simulink library "Lib_Turbo_HeatXchang_TMATS"  (R2013b)
settings: Solver=ode45  StartTime=0.0  StopTime=10.0  RelTol=1e-3
libraries: Lib_Thermo_Temp2Enth_TMATS x4, Lib_Thermo_Enth2Temp_TMATS x2, Lib_Solve_DataOut_TMATS x1
Description:
  | Thomas Modules
settings Model: Creator=jwchapm2  LastModifiedBy=jwchapm2

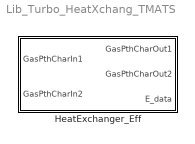
== system Lib_Turbo_HeatXchang_TMATS ==
  HeatExchanger_Eff : Subsystem  mask(T-MATS: HeatExchanger_Eff Library Block){dP1_M=0.005, dP2_M=0.005, E_M=0.5, iDesign_M=2, dQDes_M=1000, FVar_M='iDesScalars.mat', SVar_M=gcb, ENm_M='_E'}
      mask prompts: dP1_M "dP1_M - Delta Pressure for input 1 [frac lost]"; dP2_M "dP2_M - Delta Pressure for input 2 [frac lost]"; E_M "E_M - heat transfer effectiveness [frac]"; iDesign_M "iDesign_M - Design fork (0 - Enable iDes, 1 - Use iDes E, 2 - Use Input E)"; dQDes_M "dQDes_M - Delta Energy Design [BTU/sec]"; FVar_M "FVar_M - File name for iDes Variables"; SVar_M "SVar_M - iDes Variable Surname"; ENm_M "ENm_M - iDes Effectiveness variable name"
      mask help: This block simulates the performance of a heat exchanger using effectiveness-NTU method based on heat transfer efffectiveness, E.
      mask init:
      | if iDesign_M == 1
      |     load(FVar_M);
      |     E_M = eval(strcat(stripchar_TMATS(SVar_M),ENm_M));
      | end
      mask Help: web(which('Turbo_TMATS_HtXferEff.html'),'-helpbrowser')
      mask Callback iDesign_M:
      | MSK_SEC_Enables_Ides_TMATS('iDesign_M',[3],'G1')
      | MSK_SEC_Enables_Ides_TMATS('iDesign_M',[5],'G2')
      | MSK_SEC_Enables_Ides_TMATS('iDesign_M',[6 7 8],'G3')

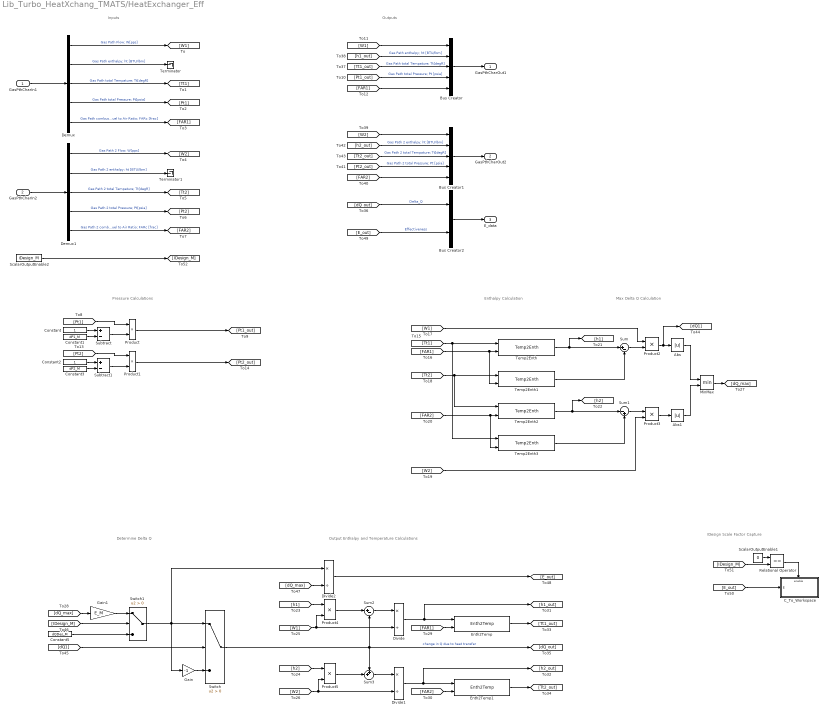
== system Lib_Turbo_HeatXchang_TMATS/HeatExchanger_Eff ==
  note: Pressure Calculations
  note: Max Delta Q Calculation
  note: Output Enthalpy and Temperature Calculations
  note: Outputs
  note: Inputs
  note: IDesign Scale Factor Capture
  note: Enthalpy Calculation
  note: Determine Delta Q
  GasPthCharIn1 : Inport
  GasPthCharIn2 : Inport  Port=2
  Abs : Abs
  Abs1 : Abs
  Bus Creator : BusCreator  Inputs=5
  Bus Creator1 : BusCreator  Inputs=5
  Bus Creator2 : BusCreator  Inputs=2
  C_To_Workspace : Subsystem
  Constant : Constant
  Constant1 : Constant  Value=dP1_M
  Constant2 : Constant
  Constant3 : Constant  Value=dP2_M
  Constant5 : Constant  Value=dQDes_M
  Demux : Demux  Outputs=5
  Demux1 : Demux  Outputs=5
  Divide : Product  Inputs=*/
  Divide1 : Product  Inputs=*/
  Divide2 : Product  Inputs=*/
  Enth2Temp : Lib_Thermo_Enth2Temp_TMATS/Enth2Temp
  Enth2Temp1 : Lib_Thermo_Enth2Temp_TMATS/Enth2Temp
  Gain : Gain  Gain=-1
  Gain1 : Gain  Gain=E_M
  MinMax : MinMax  Inputs=2
  Product : Product  RndMeth=Zero
  Product1 : Product  RndMeth=Zero
  Product{2..5} (4 alike) : Product
  Relational Operator : RelationalOperator  Operator===  OutDataTypeStr=boolean
  ScalarOutputEnable1 : Constant  Value=0
  ScalarOutputEnable2 : Constant  Value=iDesign_M
  Subtract : Sum  Inputs=+-
  Subtract1 : Sum  Inputs=+-
  Sum : Sum  Inputs=|+-
  Sum1 : Sum  Inputs=|-+
  Sum2 : Sum  Inputs=|+-
  Sum3 : Sum  Inputs=++|
  Switch : Switch  Criteria=u2 > Threshold
  Switch1 : Switch  Criteria=u2 > Threshold
  Temp2Enth{,1..3} (4 alike) : Lib_Thermo_Temp2Enth_TMATS/Temp2Enth
  Terminator : Terminator
  Terminator1 : Terminator
  GasPthCharOut1 : Outport
  GasPthCharOut2 : Outport  Port=2
  E_data : Outport  Port=3
  wires:
  Constant/1 -> Subtract/1
  Constant1/1 -> Subtract/2
  Demux/1 -> [W1]  "Gas Path Flow; W[pps]"
  Demux/5 -> [FAR1]  "Gas Path combusted Fuel to Air Ratio; FARc [frac]"
  Demux/3 -> [Tt1]  "Gas Path total Tempature; Tt[degR]"
  GasPthCharIn1/1 -> Demux/1
  Bus Creator/1 -> GasPthCharOut1/1
  Product/1 -> [Pt1_out]
  Demux/4 -> [Pt1]  "Gas Path total Pressure; Pt[psia]"
  Subtract/1 -> Product/2
  Demux/2 -> Terminator/1  "Gas Path enthalpy; ht [BTU/lbm]"
  Demux1/1 -> [W2]  "Gas Path 2 Flow; W[pps]"
  Demux1/5 -> [FAR2]  "Gas Path 2 combusted Fuel to Air Ratio; FARc [frac]"
  Demux1/3 -> [Tt2]  "Gas Path 2 total Tempature; Tt[degR]"
  GasPthCharIn2/1 -> Demux1/1
  Demux1/4 -> [Pt2]  "Gas Path 2 total Pressure; Pt[psia]"
  Demux1/2 -> Terminator1/1  "Gas Path 2 enthalpy; ht [BTU/lbm]"
  [Pt1] -> Product/1
  [Pt1_out] -> Bus Creator/4  "Gas Path total Pressure; Pt [psia]"
  [W1] -> Bus Creator/1
  [FAR1] -> Bus Creator/5
  Constant2/1 -> Subtract1/1
  Constant3/1 -> Subtract1/2
  Product1/1 -> [Pt2_out]
  Subtract1/1 -> Product1/2
  [Pt2] -> Product1/1
  [Tt1] -> Temp2Enth3/1, Temp2Enth/1
  [FAR1] -> Temp2Enth/2, Temp2Enth1/2
  [Tt2] -> Temp2Enth2/1, Temp2Enth1/1
  [FAR2] -> Temp2Enth3/2, Temp2Enth2/2
  Temp2Enth/1 -> [h1], Sum/1
  Temp2Enth2/1 -> [h2], Sum1/1
  Temp2Enth3/1 -> Sum1/2
  Temp2Enth1/1 -> Sum/2
  Sum/1 -> Product2/2
  Sum1/1 -> Product3/1
  [W1] -> Product2/1
  [W2] -> Product3/2
  Product2/1 -> [dQ1], Abs/1
  Product3/1 -> Abs1/1
  [W1] -> Product4/2, Divide/2
  [h1] -> Product4/1
  [h2] -> Product5/1
  [W2] -> Divide1/2, Product5/2
  MinMax/1 -> [dQ_max]
  Product4/1 -> Sum2/1
  Switch/1 -> [dQ_out], Sum2/2, Sum3/1  "change in Q due to heat transfer"
  Product5/1 -> Sum3/2
  Sum2/1 -> Divide/1
  Sum3/1 -> Divide1/1
  Divide/1 -> [h1_out], Enth2Temp/1
  Divide1/1 -> [h2_out], Enth2Temp1/1
  [FAR2] -> Enth2Temp1/2
  [FAR1] -> Enth2Temp/2
  Enth2Temp/1 -> [Tt1_out]
  Enth2Temp1/1 -> [Tt2_out]
  Abs/1 -> MinMax/1
  Abs1/1 -> MinMax/2
  [dQ1] -> Switch/2
  Gain/1 -> Switch/3
  [h1_out] -> Bus Creator/2  "Gas Path enthalpy; ht [BTU/lbm]"
  [Tt1_out] -> Bus Creator/3  "Gas Path total Tempature; Tt[degR]"
  [W2] -> Bus Creator1/1
  [FAR2] -> Bus Creator1/5
  [Pt2_out] -> Bus Creator1/4  "Gas Path 2 total Pressure; Pt [psia]"
  [h2_out] -> Bus Creator1/2  "Gas Path 2 enthalpy; ht [BTU/lbm]"
  [Tt2_out] -> Bus Creator1/3  "Gas Path 2 total Tempature; Tt[degR]"
  Bus Creator1/1 -> GasPthCharOut2/1
  Switch1/1 -> Gain/1, Switch/1, Divide2/1
  [dQ_out] -> Bus Creator2/1  "Delta_Q"
  Bus Creator2/1 -> E_data/1
  [IDesign_M] -> Switch1/2
  Gain1/1 -> Switch1/1
  Constant5/1 -> Switch1/3
  [dQ_max] -> Gain1/1
  Divide2/1 -> [E_out]
  [E_out] -> Bus Creator2/2  "Effectiveness"
  [dQ_max] -> Divide2/2
  [IDesign_M] -> Relational Operator/2
  ScalarOutputEnable1/1 -> Relational Operator/1
  Relational Operator/1 -> C_To_Workspace/Enable
  [E_out] -> C_To_Workspace/1(E)
  ScalarOutputEnable2/1 -> [IDesign_M]

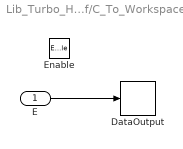
== system Lib_Turbo_HeatXchang_TMATS/HeatExchanger_Eff/C_To_Workspace ==
  E : Inport
  Enable : EnablePort
  DataOutput : Lib_Solve_DataOut_TMATS/DataOutput  FVar_M=FVar_M  Var_M=ENm_M  SVar_M=SVar_M
  wires:
  E/1 -> DataOutput/1
